simulink subsystem "LProj"  (R2020b)
settings: Solver=VariableStepAuto  StartTime=0.0  StopTime=10.0  RelTol=1e-3
settings Model: Creator=marco  LastModifiedBy=marco

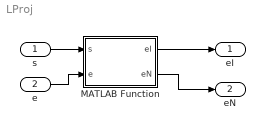
== system LProj ==
  s : Inport
  e : Inport  Port=2
  MATLAB Function : MATLAB Function  TreatAsAtomicUnit=on
  eI : Outport
  eN : Outport  Port=2
  wires:
  s/1 -> MATLAB Function/1(s)
  e/1 -> MATLAB Function/2(e)
  MATLAB Function/1(eI) -> eI/1
  MATLAB Function/2(eN) -> eN/1

== matlab function LProj/MATLAB Function ==
  data: s input; eI output; e input; eN output
function [eI, eN] = fcn(s,e)

L = computeL(s);

eI = L*pinv(L)*e;

eN = e - eI;
